simulink model "TP_Ericc3_Modele_Matlab_eleve"  (R2016b)
settings: Solver=ode3  StartTime=0.0  StopTime=2.5  FixedStep=0.01  RelTol=1e-3  EnableMultiTasking=on
values from neighbouring files (symbols this model uses):
  Cr = 0.01    [data_modele_eleve.m]
  fv = 1.17*1e-4    (= 0.000117)    [data_modele_eleve.m]
  Jeq = 2.09*1e-5    (= 2.09e-05)    [data_modele_eleve.m]
  KAN = 2*1e6/1080    (= 1851.85185185)    [data_modele_eleve.m]
  Ki = 0    [data_modele_eleve.m]
  Km = 0.043    [data_modele_eleve.m]
  Kp = 1e6    (= 1000000)    [data_modele_eleve.m]
  Kv = 0.17    [data_modele_eleve.m]
settings Model: Creator=Mathieu  LastModifiedBy=emiliendurif
settings DataIOCC: LimitDataPoints=on  SaveFormat=Array
settings OptimizationCC: LifeSpan=inf
settings DebuggingCC: SFUnexpectedBacktrackingDiag=warning  SFNoUnconditionalDefaultTransitionDiag=warning  SFExecutionAtInitializationDiag=none
settings HardwareCC: ProdBitPerPointer=32  ProdBitPerSizeT=32  ProdBitPerPtrDiffT=32  ProdLargestAtomicFloat=None  ProdIntDivRoundTo=Undefined  ProdEndianess=Unspecified  ProdWordSize=32  ProdHWDeviceType=32-bit Generic
settings ModelReferenceCC: PropagateSignalLabelsOutOfModel=off
settings GRTTargetCC: TargetLangStandard=C89/C90 (ANSI)  GeneratePreprocessorConditionals=Disable all
settings ConfigComp: CovMetricSettings=dw  CovHtmlReporting=on  CovSaveCumulativeToWorkspaceVar=on  CovSaveSingleToWorkspaceVar=on  CovExternalEMLEnable=off

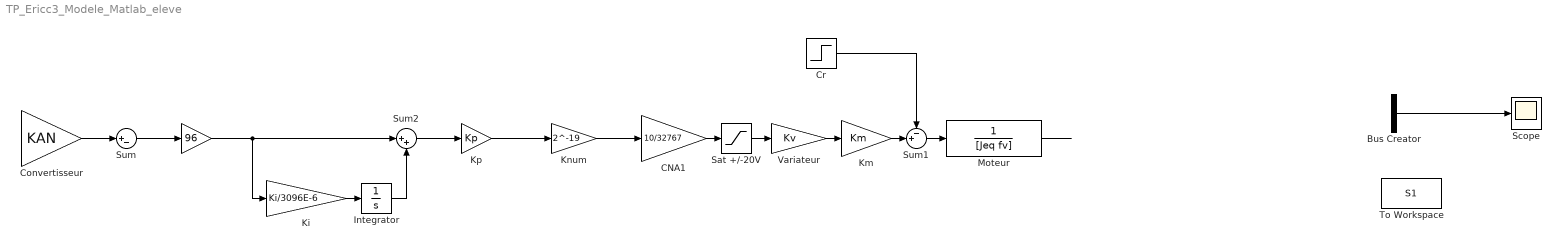
== system TP_Ericc3_Modele_Matlab_eleve ==
  " " : Gain  Gain=96
  Bus Creator : BusCreator  Inputs=2
  CNA1 : Gain  Gain=10/32767
  Convertisseur : Gain  Gain=KAN
  Cr : Step  Time=0  After=Cr  SampleTime=0
  Integrator : Integrator
  Ki : Gain  Gain=Ki/3096E-6
  Km : Gain  Gain=Km
  Knum : Gain  Gain=2^-19
  Kp : Gain  Gain=Kp
  Moteur : TransferFcn  Denominator=[Jeq fv]
  Sat +/-20V : Saturate  UpperLimit=10  LowerLimit=-10
  Scope : Scope
  Sum : Sum  Inputs=|+-
  Sum1 : Sum  Inputs=-+|
  Sum2 : Sum  Inputs=|++
  To Workspace : ToWorkspace  VariableName=S1  SaveFormat=Timeseries  SampleTime=-1
  "Variateur " : Gain  Gain=Kv
  wires:
  Convertisseur/1 -> Sum/1
  ? -> Bus Creator/1, Convertisseur/1
  "Variateur "/1 -> Km/1
  Km/1 -> Sum1/2
  Moteur/1 -> ?
  ? -> To Workspace/1, Bus Creator/2
  Bus Creator/1 -> Scope/1
  Cr/1 -> Sum1/1
  Sum/1 -> " "/1
  " "/1 -> Ki/1, Sum2/1
  Sum2/1 -> Kp/1
  Integrator/1 -> Sum2/2
  Ki/1 -> Integrator/1
  Sum1/1 -> Moteur/1
  Knum/1 -> CNA1/1
  CNA1/1 -> Sat +/-20V/1
  Sat +/-20V/1 -> "Variateur "/1
  Kp/1 -> Knum/1
